simulink model "controlLoopDebuging"  (R2020a)
settings: Solver=FixedStepAuto  StartTime=0.0  StopTime=inf  FixedStep=.005  RelTol=1e-3
undefined symbols (not defined in the file or in its folder): DiscIntNeverNeededParam
libraries: simulink x17
settings Model: Creator=Hiwi  LastModifiedBy=Hiwi

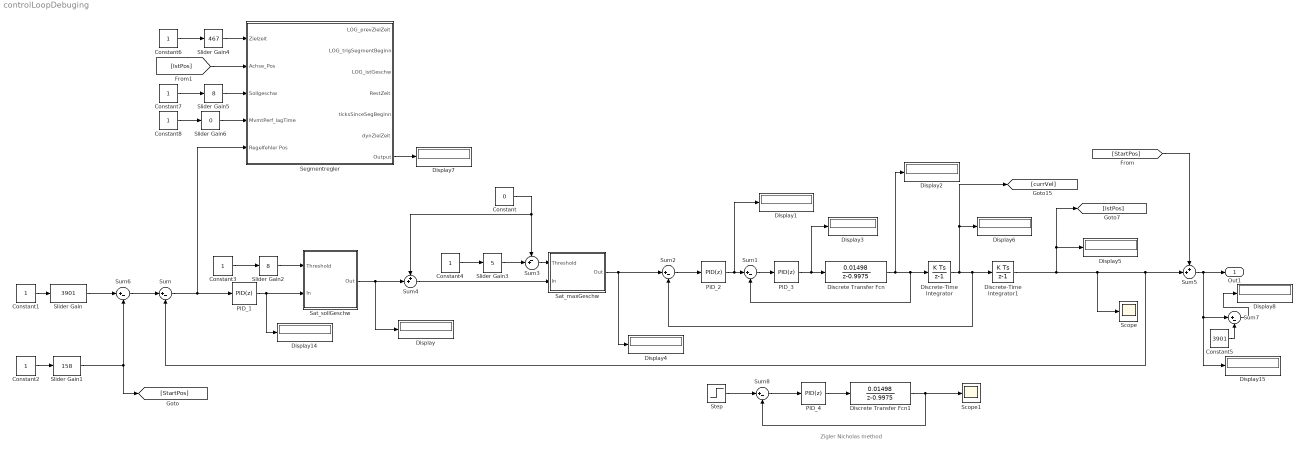
== system controlLoopDebuging ==
  note: Zigler Nicholas method
  Constant : Constant  Value=0
  Constant{1..4,6..8} (7 alike) : Constant
  Constant5 : Constant  Value=3901
  Discrete Transfer Fcn : DiscreteTransferFcn  Numerator=0.01498  Denominator=[1 -0.9975]
  Discrete Transfer Fcn1 : DiscreteTransferFcn  Numerator=0.01498  Denominator=[1 -0.9975]
  Discrete-Time Integrator : DiscreteIntegrator  SampleTime=-1  ICPrevOutput=DiscIntNeverNeededParam  ICPrevScaledInput=DiscIntNeverNeededParam
  Discrete-Time Integrator1 : DiscreteIntegrator  SampleTime=-1  ICPrevOutput=DiscIntNeverNeededParam  ICPrevScaledInput=DiscIntNeverNeededParam
  Display{,1..8,14..15} (11 alike) : Display
  PID_1 : simulink/Continuous/PID Controller  Controller=PID  Form=Parallel  TimeDomain=Discrete-time  UseExternalTs=off  SampleTime=-1  IntegratorMethod=Forward Euler  FilterMethod=Forward Euler  ControllerParametersSource=internal  P=20  I=0  D=0  UseFilter=on  N=100  TunerSelectOption=Transfer Function Based (PID Tuner App)  InitialConditionSource=internal  InitialConditionForIntegrator=0  InitialConditionForFilter=0  DifferentiatorICPrevScaledInput=0  ExternalReset=none  TrackingMode=off  Kt=1  LimitOutput=off  UpperSaturationLimit=inf  LowerSaturationLimit=-inf  LinearizeAsGain=off  AntiWindupMode=none  Kb=1  POutMin=[]  POutMax=[]  IOutMin=[]  IOutMax=[]  DOutMin=[]  DOutMax=[]  NOutMin=[]  NOutMax=[]  SumOutMin=[]  SumOutMax=[]  SaturationOutMin=[]  SaturationOutMax=[]  PParamMin=[]  PParamMax=[]  IParamMin=[]  IParamMax=[]  DParamMin=[]  DParamMax=[]  NParamMin=[]  NParamMax=[]  KbParamMin=[]  KbParamMax=[]  KtParamMin=[]  KtParamMax=[]  KbOutMin=[]  KbOutMax=[]  KtOutMin=[]  KtOutMax=[]  IntegratorOutMin=[]  IntegratorOutMax=[]  FilterOutMin=[]  FilterOutMax=[]  SumI1OutMin=[]  SumI1OutMax=[]  SumI2OutMin=[]  SumI2OutMax=[]  SumI3OutMin=[]  SumI3OutMax=[]  SumI4OutMin=[]  SumI4OutMax=[]  SumDOutMin=[]  SumDOutMax=[]  DifferentiatorOutMin=[]  DifferentiatorOutMax=[]  FilterDiffOutCoefMin=[]  FilterDiffOutCoefMax=[]  ReciprocalOutMin=[]  ReciprocalOutMax=[]  SumDenOutMin=[]  SumDenOutMax=[]  SumNumOutMin=[]  SumNumOutMax=[]  DivideOutMin=[]  DivideOutMax=[]  UdiffTsProdOutMin=[]  UdiffTsProdOutMax=[]  NTsProdOutMin=[]  NTsProdOutMax=[]  UintegralTsProdOutMin=[]  UintegralTsProdOutMax=[]  UngainTsProdOutMin=[]  UngainTsProdOutMax=[]  IntegratorContinuousStateAttributes=''  IntegratorStateMustResolveToSignalObject=off  IntegratorRTWStateStorageClass=Auto  FilterContinuousStateAttributes=''  FilterStateMustResolveToSignalObject=off  FilterRTWStateStorageClass=Auto  ParallelPVariant=InternalParameters  IdealPVariant=Disabled  IVariant=InternalParameters  DVariant=InternalParameters  IntegratorVariant=Discrete  SatVariant=Disabled  AWVariant=Passthrough  PCopyVariant=Disabled  TRVariant=Disabled  FdbkBlocksVariant=Forward  IdealPFdbkVariant=Disabled  SatFdbkVariant=Disabled  DerivativeFilterVariant=ForwardEulerFilter  NVariant=InternalParameters  NCopyVariant=Disabled  FilterICVariant=InternalICsFilter  IntegratorICVariant=InternalICs  ExternalResetVariant=Disabled  TRSumVariant=Passthrough  SumFdbkVariant=Disabled  SumVariant=Sum_PID  TsampFilterVariant=InternalTs  TsampNgainVariant=Passthrough  TsampIntegralVariant=Passthrough
  PID_2 : simulink/Continuous/PID Controller  Controller=PID  Form=Parallel  TimeDomain=Discrete-time  UseExternalTs=off  SampleTime=-1  IntegratorMethod=Forward Euler  FilterMethod=Forward Euler  ControllerParametersSource=internal  P=20  I=1  D=0  UseFilter=on  N=100  TunerSelectOption=Transfer Function Based (PID Tuner App)  InitialConditionSource=internal  InitialConditionForIntegrator=0  InitialConditionForFilter=0  DifferentiatorICPrevScaledInput=0  ExternalReset=none  TrackingMode=off  Kt=1  LimitOutput=off  UpperSaturationLimit=inf  LowerSaturationLimit=-inf  LinearizeAsGain=off  AntiWindupMode=none  Kb=1  POutMin=[]  POutMax=[]  IOutMin=[]  IOutMax=[]  DOutMin=[]  DOutMax=[]  NOutMin=[]  NOutMax=[]  SumOutMin=[]  SumOutMax=[]  SaturationOutMin=[]  SaturationOutMax=[]  PParamMin=[]  PParamMax=[]  IParamMin=[]  IParamMax=[]  DParamMin=[]  DParamMax=[]  NParamMin=[]  NParamMax=[]  KbParamMin=[]  KbParamMax=[]  KtParamMin=[]  KtParamMax=[]  KbOutMin=[]  KbOutMax=[]  KtOutMin=[]  KtOutMax=[]  IntegratorOutMin=[]  IntegratorOutMax=[]  FilterOutMin=[]  FilterOutMax=[]  SumI1OutMin=[]  SumI1OutMax=[]  SumI2OutMin=[]  SumI2OutMax=[]  SumI3OutMin=[]  SumI3OutMax=[]  SumI4OutMin=[]  SumI4OutMax=[]  SumDOutMin=[]  SumDOutMax=[]  DifferentiatorOutMin=[]  DifferentiatorOutMax=[]  FilterDiffOutCoefMin=[]  FilterDiffOutCoefMax=[]  ReciprocalOutMin=[]  ReciprocalOutMax=[]  SumDenOutMin=[]  SumDenOutMax=[]  SumNumOutMin=[]  SumNumOutMax=[]  DivideOutMin=[]  DivideOutMax=[]  UdiffTsProdOutMin=[]  UdiffTsProdOutMax=[]  NTsProdOutMin=[]  NTsProdOutMax=[]  UintegralTsProdOutMin=[]  UintegralTsProdOutMax=[]  UngainTsProdOutMin=[]  UngainTsProdOutMax=[]  IntegratorContinuousStateAttributes=''  IntegratorStateMustResolveToSignalObject=off  IntegratorRTWStateStorageClass=Auto  FilterContinuousStateAttributes=''  FilterStateMustResolveToSignalObject=off  FilterRTWStateStorageClass=Auto  ParallelPVariant=InternalParameters  IdealPVariant=Disabled  IVariant=InternalParameters  DVariant=InternalParameters  IntegratorVariant=Discrete  SatVariant=Disabled  AWVariant=Passthrough  PCopyVariant=Disabled  TRVariant=Disabled  FdbkBlocksVariant=Forward  IdealPFdbkVariant=Disabled  SatFdbkVariant=Disabled  DerivativeFilterVariant=ForwardEulerFilter  NVariant=InternalParameters  NCopyVariant=Disabled  FilterICVariant=InternalICsFilter  IntegratorICVariant=InternalICs  ExternalResetVariant=Disabled  TRSumVariant=Passthrough  SumFdbkVariant=Disabled  SumVariant=Sum_PID  TsampFilterVariant=InternalTs  TsampNgainVariant=Passthrough  TsampIntegralVariant=Passthrough
  PID_3 : simulink/Continuous/PID Controller  Controller=PID  Form=Parallel  TimeDomain=Discrete-time  UseExternalTs=off  SampleTime=-1  IntegratorMethod=Forward Euler  FilterMethod=Forward Euler  ControllerParametersSource=internal  P=20  I=1  D=0  UseFilter=on  N=100  TunerSelectOption=Transfer Function Based (PID Tuner App)  InitialConditionSource=internal  InitialConditionForIntegrator=0  InitialConditionForFilter=0  DifferentiatorICPrevScaledInput=0  ExternalReset=none  TrackingMode=off  Kt=1  LimitOutput=off  UpperSaturationLimit=inf  LowerSaturationLimit=-inf  LinearizeAsGain=off  AntiWindupMode=none  Kb=1  POutMin=[]  POutMax=[]  IOutMin=[]  IOutMax=[]  DOutMin=[]  DOutMax=[]  NOutMin=[]  NOutMax=[]  SumOutMin=[]  SumOutMax=[]  SaturationOutMin=[]  SaturationOutMax=[]  PParamMin=[]  PParamMax=[]  IParamMin=[]  IParamMax=[]  DParamMin=[]  DParamMax=[]  NParamMin=[]  NParamMax=[]  KbParamMin=[]  KbParamMax=[]  KtParamMin=[]  KtParamMax=[]  KbOutMin=[]  KbOutMax=[]  KtOutMin=[]  KtOutMax=[]  IntegratorOutMin=[]  IntegratorOutMax=[]  FilterOutMin=[]  FilterOutMax=[]  SumI1OutMin=[]  SumI1OutMax=[]  SumI2OutMin=[]  SumI2OutMax=[]  SumI3OutMin=[]  SumI3OutMax=[]  SumI4OutMin=[]  SumI4OutMax=[]  SumDOutMin=[]  SumDOutMax=[]  DifferentiatorOutMin=[]  DifferentiatorOutMax=[]  FilterDiffOutCoefMin=[]  FilterDiffOutCoefMax=[]  ReciprocalOutMin=[]  ReciprocalOutMax=[]  SumDenOutMin=[]  SumDenOutMax=[]  SumNumOutMin=[]  SumNumOutMax=[]  DivideOutMin=[]  DivideOutMax=[]  UdiffTsProdOutMin=[]  UdiffTsProdOutMax=[]  NTsProdOutMin=[]  NTsProdOutMax=[]  UintegralTsProdOutMin=[]  UintegralTsProdOutMax=[]  UngainTsProdOutMin=[]  UngainTsProdOutMax=[]  IntegratorContinuousStateAttributes=''  IntegratorStateMustResolveToSignalObject=off  IntegratorRTWStateStorageClass=Auto  FilterContinuousStateAttributes=''  FilterStateMustResolveToSignalObject=off  FilterRTWStateStorageClass=Auto  ParallelPVariant=InternalParameters  IdealPVariant=Disabled  IVariant=InternalParameters  DVariant=InternalParameters  IntegratorVariant=Discrete  SatVariant=Disabled  AWVariant=Passthrough  PCopyVariant=Disabled  TRVariant=Disabled  FdbkBlocksVariant=Forward  IdealPFdbkVariant=Disabled  SatFdbkVariant=Disabled  DerivativeFilterVariant=ForwardEulerFilter  NVariant=InternalParameters  NCopyVariant=Disabled  FilterICVariant=InternalICsFilter  IntegratorICVariant=InternalICs  ExternalResetVariant=Disabled  TRSumVariant=Passthrough  SumFdbkVariant=Disabled  SumVariant=Sum_PID  TsampFilterVariant=InternalTs  TsampNgainVariant=Passthrough  TsampIntegralVariant=Passthrough
  PID_4 : simulink/Continuous/PID Controller  Controller=PID  Form=Parallel  TimeDomain=Discrete-time  UseExternalTs=off  SampleTime=-1  IntegratorMethod=Forward Euler  FilterMethod=Forward Euler  ControllerParametersSource=internal  P=20  I=0  D=0  UseFilter=on  N=0  TunerSelectOption=Transfer Function Based (PID Tuner App)  InitialConditionSource=internal  InitialConditionForIntegrator=0  InitialConditionForFilter=0  DifferentiatorICPrevScaledInput=0  ExternalReset=none  TrackingMode=off  Kt=1  LimitOutput=off  UpperSaturationLimit=inf  LowerSaturationLimit=-inf  LinearizeAsGain=off  AntiWindupMode=none  Kb=1  POutMin=[]  POutMax=[]  IOutMin=[]  IOutMax=[]  DOutMin=[]  DOutMax=[]  NOutMin=[]  NOutMax=[]  SumOutMin=[]  SumOutMax=[]  SaturationOutMin=[]  SaturationOutMax=[]  PParamMin=[]  PParamMax=[]  IParamMin=[]  IParamMax=[]  DParamMin=[]  DParamMax=[]  NParamMin=[]  NParamMax=[]  KbParamMin=[]  KbParamMax=[]  KtParamMin=[]  KtParamMax=[]  KbOutMin=[]  KbOutMax=[]  KtOutMin=[]  KtOutMax=[]  IntegratorOutMin=[]  IntegratorOutMax=[]  FilterOutMin=[]  FilterOutMax=[]  SumI1OutMin=[]  SumI1OutMax=[]  SumI2OutMin=[]  SumI2OutMax=[]  SumI3OutMin=[]  SumI3OutMax=[]  SumI4OutMin=[]  SumI4OutMax=[]  SumDOutMin=[]  SumDOutMax=[]  DifferentiatorOutMin=[]  DifferentiatorOutMax=[]  FilterDiffOutCoefMin=[]  FilterDiffOutCoefMax=[]  ReciprocalOutMin=[]  ReciprocalOutMax=[]  SumDenOutMin=[]  SumDenOutMax=[]  SumNumOutMin=[]  SumNumOutMax=[]  DivideOutMin=[]  DivideOutMax=[]  UdiffTsProdOutMin=[]  UdiffTsProdOutMax=[]  NTsProdOutMin=[]  NTsProdOutMax=[]  UintegralTsProdOutMin=[]  UintegralTsProdOutMax=[]  UngainTsProdOutMin=[]  UngainTsProdOutMax=[]  IntegratorContinuousStateAttributes=''  IntegratorStateMustResolveToSignalObject=off  IntegratorRTWStateStorageClass=Auto  FilterContinuousStateAttributes=''  FilterStateMustResolveToSignalObject=off  FilterRTWStateStorageClass=Auto  ParallelPVariant=InternalParameters  IdealPVariant=Disabled  IVariant=InternalParameters  DVariant=InternalParameters  IntegratorVariant=Discrete  SatVariant=Disabled  AWVariant=Passthrough  PCopyVariant=Disabled  TRVariant=Disabled  FdbkBlocksVariant=Forward  IdealPFdbkVariant=Disabled  SatFdbkVariant=Disabled  DerivativeFilterVariant=ForwardEulerFilter  NVariant=InternalParameters  NCopyVariant=Disabled  FilterICVariant=InternalICsFilter  IntegratorICVariant=InternalICs  ExternalResetVariant=Disabled  TRSumVariant=Passthrough  SumFdbkVariant=Disabled  SumVariant=Sum_PID  TsampFilterVariant=InternalTs  TsampNgainVariant=Passthrough  TsampIntegralVariant=Passthrough
  Sat_maxGeschw : Subsystem
  Sat_sollGeschw : Subsystem
  Scope : Scope
  Scope1 : Scope
  Segmentregler : Subsystem
  Slider Gain : simulink/Math Operations/Slider Gain  gain=3901  low=0  high=10000
  Slider Gain1 : simulink/Math Operations/Slider Gain  gain=158  low=0  high=10000
  Slider Gain2 : simulink/Math Operations/Slider Gain  gain=8  low=0  high=100
  Slider Gain3 : simulink/Math Operations/Slider Gain  gain=5  low=0  high=10
  Slider Gain4 : simulink/Math Operations/Slider Gain  gain=467  low=0  high=1000
  Slider Gain5 : simulink/Math Operations/Slider Gain  gain=8  low=0  high=100
  Slider Gain6 : simulink/Math Operations/Slider Gain  gain=0  low=0  high=100
  Step : Step  SampleTime=0
  Sum{,1..2,6..8} (6 alike) : Sum  Inputs=|+-
  Sum3 : Sum  Inputs=-+|
  Sum4 : Sum  Inputs=++|
  Sum5 : Sum  Inputs=++|
  Out1 : Outport  VectorParamsAs1DForOutWhenUnconnected=off
  wires:
  Sum/1 -> Segmentregler/5(Regelfehler Pos), PID_1/1
  Slider Gain3/1 -> Sum3/2
  Sat_maxGeschw/1(Out) -> Display4/1, Sum2/1
  Sum2/1 -> PID_2/1
  Discrete-Time Integrator/1 -> Display6/1, [currVel], Discrete-Time Integrator1/1, Sum2/2
  Sum3/1 -> Sat_maxGeschw/1(Threshold)
  PID_1/1 -> Display14/1, Sat_sollGeschw/2(In)
  [StartPos] -> Sum5/1
  PID_2/1 -> Display1/1, Sum1/1
  Sum1/1 -> PID_3/1
  Sum5/1 -> Out1/1, Sum7/1, Display15/1
  Sat_sollGeschw/1(Out) -> Display/1, Sum4/2
  Discrete Transfer Fcn/1 -> Display2/1, Discrete-Time Integrator/1, Sum1/2
  Discrete-Time Integrator1/1 -> Display5/1, [IstPos], Scope/1, Sum5/2, Sum/2
  PID_3/1 -> Display3/1, Discrete Transfer Fcn/1
  Sum4/1 -> Sat_maxGeschw/2(In)
  Sum6/1 -> Sum/1
  Slider Gain/1 -> Sum6/1
  Constant1/1 -> Slider Gain/1
  Constant2/1 -> Slider Gain1/1
  Slider Gain2/1 -> Sat_sollGeschw/1(Threshold)
  Constant3/1 -> Slider Gain2/1
  Constant4/1 -> Slider Gain3/1
  Segmentregler/7(Output) -> Display7/1
  Slider Gain1/1 -> [StartPos], Sum6/2
  Slider Gain4/1 -> Segmentregler/1(Zielzeit)
  Constant6/1 -> Slider Gain4/1
  [IstPos] -> Segmentregler/2(Achse_Pos)
  Slider Gain5/1 -> Segmentregler/3(Sollgeschw)
  Constant7/1 -> Slider Gain5/1
  Constant8/1 -> Slider Gain6/1
  Slider Gain6/1 -> Segmentregler/4(MvmtPerf_lagTime)
  Constant/1 -> Sum4/1, Sum3/1
  Constant5/1 -> Sum7/2
  Sum7/1 -> Display8/1
  PID_4/1 -> Discrete Transfer Fcn1/1
  Step/1 -> Sum8/1
  Sum8/1 -> PID_4/1
  Discrete Transfer Fcn1/1 -> Scope1/1, Sum8/2

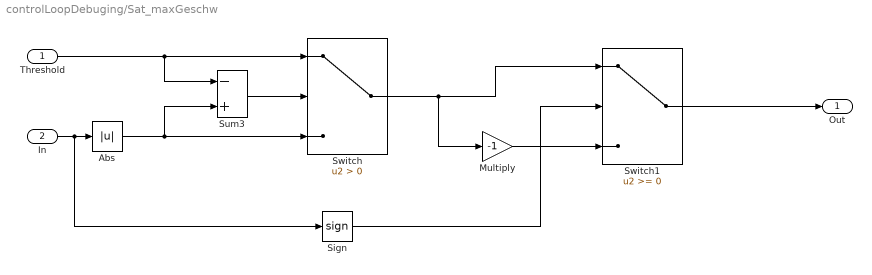
== system controlLoopDebuging/Sat_maxGeschw ==
  Threshold : Inport
  In : Inport  Port=2
  Abs : Abs
  Multiply : Gain  Gain=-1
  Sign : Signum
  Sum3 : Sum  Inputs=-+
  Switch : Switch  Criteria=u2 > Threshold
  Switch1 : Switch
  Out : Outport  VectorParamsAs1DForOutWhenUnconnected=off
  wires:
  Switch1/1 -> Out/1
  Multiply/1 -> Switch1/3
  Switch/1 -> Switch1/1, Multiply/1
  Sign/1 -> Switch1/2
  In/1 -> Abs/1, Sign/1
  Abs/1 -> Switch/3, Sum3/2
  Threshold/1 -> Sum3/1, Switch/1
  Sum3/1 -> Switch/2

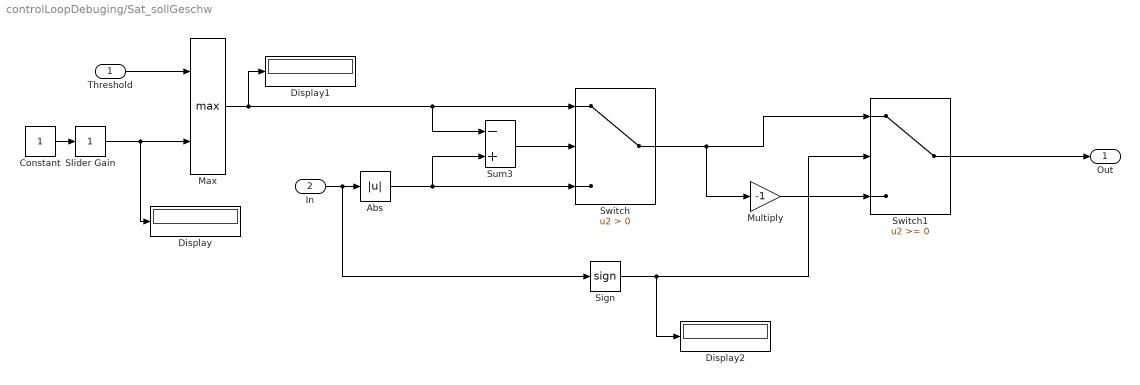
== system controlLoopDebuging/Sat_sollGeschw ==
  Threshold : Inport
  In : Inport  Port=2
  Abs : Abs
  Constant : Constant
  Display : Display
  Display1 : Display
  Display2 : Display
  Max : MinMax  Function=max  Inputs=2
  Multiply : Gain  Gain=-1
  Sign : Signum
  Slider Gain : simulink/Math Operations/Slider Gain  gain=1  low=0  high=100
  Sum3 : Sum  Inputs=-+
  Switch : Switch  Criteria=u2 > Threshold
  Switch1 : Switch
  Out : Outport  VectorParamsAs1DForOutWhenUnconnected=off
  wires:
  Sum3/1 -> Switch/2
  Max/1 -> Display1/1, Switch/1, Sum3/1
  Abs/1 -> Sum3/2, Switch/3
  In/1 -> Sign/1, Abs/1
  Sign/1 -> Display2/1, Switch1/2
  Switch/1 -> Multiply/1, Switch1/1
  Multiply/1 -> Switch1/3
  Switch1/1 -> Out/1
  Threshold/1 -> Max/1
  Slider Gain/1 -> Display/1, Max/2
  Constant/1 -> Slider Gain/1

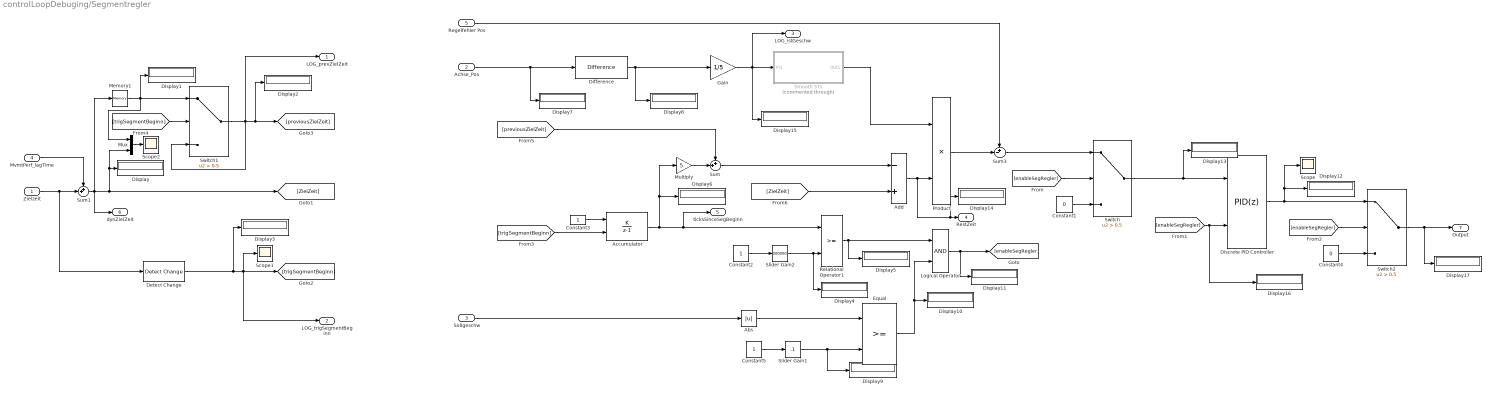
== system controlLoopDebuging/Segmentregler ==
  Zielzeit : Inport
  Achse_Pos : Inport  Port=2
  Sollgeschw : Inport  Port=3
  MvmtPerf_lagTime : Inport  Port=4
  Regelfehler Pos : Inport  Port=5
  Abs : Abs
  Accumulator : DiscreteIntegrator  IntegratorMethod=Accumulation: Forward Euler  gainval=1  ExternalReset=rising  SampleTime=-1  ICPrevOutput=DiscIntNeverNeededParam  ICPrevScaledInput=DiscIntNeverNeededParam
  Add : Sum  Inputs=-+
  Constant1 : Constant  Value=0
  Constant2 : Constant
  Constant3 : Constant
  Constant4 : Constant  Value=0
  Constant5 : Constant
  Detect Change : simulink/Logic and Bit Operations/Detect Change  vinit=0  OutDataTypeStr=boolean
  Difference : simulink/Discrete/Difference  ICPrevInput=0.0  OutMin=[]  OutMax=[]  OutDataType=fixdt(1, 16)  OutScaling=2^-10  DoSatur=off
  Discrete PID Controller : simulink/Continuous/PID Controller  Controller=PID  Form=Parallel  TimeDomain=Discrete-time  UseExternalTs=off  SampleTime=-1  IntegratorMethod=Forward Euler  FilterMethod=Forward Euler  ControllerParametersSource=internal  P=0  I=1  D=0  UseFilter=on  N=100  TunerSelectOption=Transfer Function Based (PID Tuner App)  InitialConditionSource=internal  InitialConditionForIntegrator=0  InitialConditionForFilter=0  DifferentiatorICPrevScaledInput=0  ExternalReset=falling  TrackingMode=off  Kt=1  LimitOutput=off  UpperSaturationLimit=inf  LowerSaturationLimit=-inf  LinearizeAsGain=off  AntiWindupMode=none  Kb=1  POutMin=[]  POutMax=[]  IOutMin=[]  IOutMax=[]  DOutMin=[]  DOutMax=[]  NOutMin=[]  NOutMax=[]  SumOutMin=[]  SumOutMax=[]  SaturationOutMin=[]  SaturationOutMax=[]  PParamMin=[]  PParamMax=[]  IParamMin=[]  IParamMax=[]  DParamMin=[]  DParamMax=[]  NParamMin=[]  NParamMax=[]  KbParamMin=[]  KbParamMax=[]  KtParamMin=[]  KtParamMax=[]  KbOutMin=[]  KbOutMax=[]  KtOutMin=[]  KtOutMax=[]  IntegratorOutMin=[]  IntegratorOutMax=[]  FilterOutMin=[]  FilterOutMax=[]  SumI1OutMin=[]  SumI1OutMax=[]  SumI2OutMin=[]  SumI2OutMax=[]  SumI3OutMin=[]  SumI3OutMax=[]  SumI4OutMin=[]  SumI4OutMax=[]  SumDOutMin=[]  SumDOutMax=[]  DifferentiatorOutMin=[]  DifferentiatorOutMax=[]  FilterDiffOutCoefMin=[]  FilterDiffOutCoefMax=[]  ReciprocalOutMin=[]  ReciprocalOutMax=[]  SumDenOutMin=[]  SumDenOutMax=[]  SumNumOutMin=[]  SumNumOutMax=[]  DivideOutMin=[]  DivideOutMax=[]  UdiffTsProdOutMin=[]  UdiffTsProdOutMax=[]  NTsProdOutMin=[]  NTsProdOutMax=[]  UintegralTsProdOutMin=[]  UintegralTsProdOutMax=[]  UngainTsProdOutMin=[]  UngainTsProdOutMax=[]  IntegratorContinuousStateAttributes=''  IntegratorStateMustResolveToSignalObject=off  IntegratorRTWStateStorageClass=Auto  FilterContinuousStateAttributes=''  FilterStateMustResolveToSignalObject=off  FilterRTWStateStorageClass=Auto  ParallelPVariant=InternalParameters  IdealPVariant=Disabled  IVariant=InternalParameters  DVariant=InternalParameters  IntegratorVariant=Discrete  SatVariant=Disabled  AWVariant=Passthrough  PCopyVariant=Disabled  TRVariant=Disabled  FdbkBlocksVariant=Forward  IdealPFdbkVariant=Disabled  SatFdbkVariant=Disabled  DerivativeFilterVariant=ForwardEulerFilter  NVariant=InternalParameters  NCopyVariant=Disabled  FilterICVariant=InternalICsFilter  IntegratorICVariant=InternalICs  ExternalResetVariant=ExternalReset  TRSumVariant=Passthrough  SumFdbkVariant=Disabled  SumVariant=Sum_PID  TsampFilterVariant=InternalTs  TsampNgainVariant=Passthrough  TsampIntegralVariant=Passthrough
  Display{,1..17} (18 alike) : Display
  Equal : RelationalOperator  OutDataTypeStr=boolean  RndMeth=Simplest
  Gain : Gain  Gain=1/5
  Logical Operator : Logic  AllPortsSameDT=off  OutDataTypeStr=boolean
  Memory1 : Memory
  Multiply : Gain  Gain=5
  Mux : Mux  Inputs=2
  Product : Product
  Relational Operator1 : RelationalOperator  OutDataTypeStr=boolean  RndMeth=Simplest
  Scope : Scope
  Scope1 : Scope
  Scope2 : Scope
  Slider Gain1 : simulink/Math Operations/Slider Gain  gain=.1  low=0  high=100
  Slider Gain2 : simulink/Math Operations/Slider Gain  gain=300000  low=0  high=10000000
  Smooth 5Ts : Subsystem  Commented=through
  Sum : Sum  Inputs=++|
  Sum1 : Sum  Inputs=++|
  Sum3 : Sum  Inputs=+-|
  Switch : Switch  Criteria=u2 > Threshold  Threshold=0.5
  Switch1 : Switch  Criteria=u2 > Threshold  Threshold=0.5
  Switch2 : Switch  Criteria=u2 > Threshold  Threshold=0.5
  LOG_prevZielZeit : Outport  VectorParamsAs1DForOutWhenUnconnected=off
  LOG_trigSegmentBeginn : Outport  Port=2  VectorParamsAs1DForOutWhenUnconnected=off
  LOG_istGeschw : Outport  Port=3  VectorParamsAs1DForOutWhenUnconnected=off
  RestZeit : Outport  Port=4  VectorParamsAs1DForOutWhenUnconnected=off
  ticksSinceSegBeginn : Outport  Port=5  VectorParamsAs1DForOutWhenUnconnected=off
  dynZielZeit : Outport  Port=6  VectorParamsAs1DForOutWhenUnconnected=off
  Output : Outport  Port=7  VectorParamsAs1DForOutWhenUnconnected=off
  wires:
  Constant3/1 -> Accumulator/1
  Difference/1 -> Display8/1, Gain/1
  Sum3/1 -> Switch/1
  Switch/1 -> Display13/1, Discrete PID Controller/1
  Sum/1 -> Add/1
  Relational Operator1/1 -> Display5/1, Logical Operator/1
  Add/1 -> Display14/1, RestZeit/1, Product/2
  Slider Gain2/1 -> Display4/1, Relational Operator1/2
  Achse_Pos/1 -> Display7/1, Difference/1
  Discrete PID Controller/1 -> Display12/1, Scope/1, Switch2/1
  Constant1/1 -> Switch/3
  Constant4/1 -> Switch2/3
  Product/1 -> Sum3/2
  Regelfehler Pos/1 -> Sum3/1
  Switch2/1 -> Display17/1, Output/1
  Logical Operator/1 -> Display11/1, [enableSegRegler]
  [enableSegRegler] -> Switch/2
  [enableSegRegler] -> Switch2/2
  Sollgeschw/1 -> Abs/1
  Slider Gain1/1 -> Display9/1, Equal/2
  Equal/1 -> Display10/1, Logical Operator/2
  Sum1/1 -> Memory1/1, Mux/2, Display/1, [ZielZeit], dynZielZeit/1
  Gain/1 -> Display15/1, LOG_istGeschw/1, Smooth 5Ts/1(In1)
  Detect Change/1 -> Display3/1, Scope1/1, LOG_trigSegmentBeginn/1, [trigSegmentBeginn]
  [trigSegmentBeginn] -> Switch1/2
  Switch1/1 -> Display2/1, [previousZielZeit], Switch1/3, LOG_prevZielZeit/1
  [previousZielZeit] -> Sum/1
  Smooth 5Ts/1(Out1) -> Product/1
  Multiply/1 -> Sum/2
  [ZielZeit] -> Add/2
  Abs/1 -> Equal/1
  Zielzeit/1 -> Detect Change/1, Sum1/2
  MvmtPerf_lagTime/1 -> Sum1/1
  Accumulator/1 -> Display6/1, Multiply/1, ticksSinceSegBeginn/1, Relational Operator1/1
  [trigSegmentBeginn] -> Accumulator/2
  [enableSegRegler] -> Display16/1, Discrete PID Controller/2
  Mux/1 -> Scope2/1
  Memory1/1 -> Mux/1, Display1/1, Switch1/1
  Constant2/1 -> Slider Gain2/1
  Constant5/1 -> Slider Gain1/1

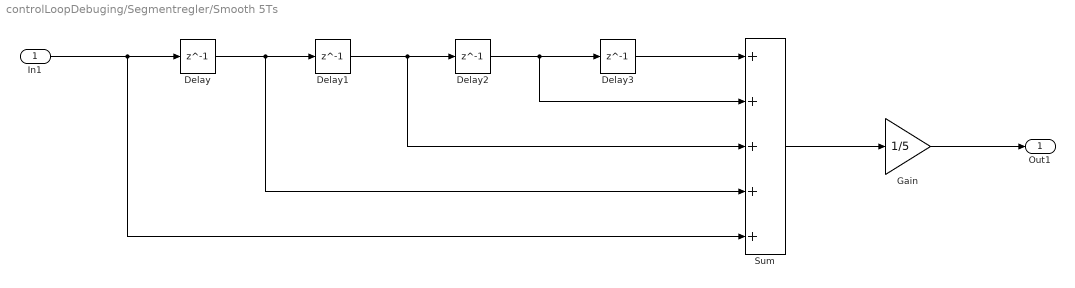
== system controlLoopDebuging/Segmentregler/Smooth 5Ts ==
  In1 : Inport
  Delay{,1..3} (4 alike) : Delay  DelayLength=1
  Gain : Gain  Gain=1/5
  Sum : Sum  Inputs=+++++
  Out1 : Outport  VectorParamsAs1DForOutWhenUnconnected=off
  wires:
  In1/1 -> Sum/5, Delay/1
  Delay/1 -> Sum/4, Delay1/1
  Delay1/1 -> Sum/3, Delay2/1
  Delay2/1 -> Sum/2, Delay3/1
  Delay3/1 -> Sum/1
  Sum/1 -> Gain/1
  Gain/1 -> Out1/1
